simulink model "psk"  (R2023b)
settings: Solver=ode3  StartTime=0.0  StopTime=10.0  FixedStep=0.01  RelTol=1e-3
settings Model: Creator=ASUS  LastModifiedBy=ASUS

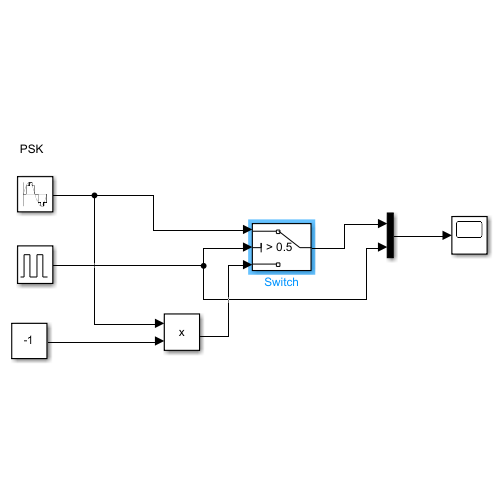
[thumbnail: Simulink's stored preview of the top-level diagram]
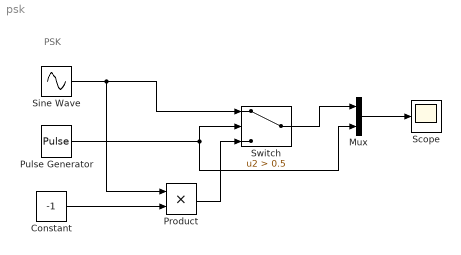
== system psk ==
  note: PSK
  Constant : Constant  Value=-1
  Mux : Mux  Inputs=2
  Product : Product
  Pulse Generator : DiscretePulseGenerator  PulseType=Time based  PulseWidth=50
  Scope : Scope
  Sine Wave : Sin  Frequency=2*pi*2  SampleTime=0.01
  Switch : Switch  Criteria=u2 > Threshold  Threshold=0.5  SaturateOnIntegerOverflow=off  InputSameDT=off
  wires:
  Sine Wave/1 -> Product/1, Switch/1
  Pulse Generator/1 -> Switch/2, Mux/2
  Constant/1 -> Product/2
  Product/1 -> Switch/3
  Mux/1 -> Scope/1
  Switch/1 -> Mux/1
